simulink model "sampleModel1924_5_sub_sub"  (R2023a)
settings: Solver=VariableStepAuto  StartTime=0.0  StopTime=10.0  RelTol=1e-3
libraries: hdlsllib x5, simulink x2
settings Model: Creator=user1  LastModifiedBy=user1
settings OptimizationCC: BlockReduction=off  ConditionallyExecuteInputs=off

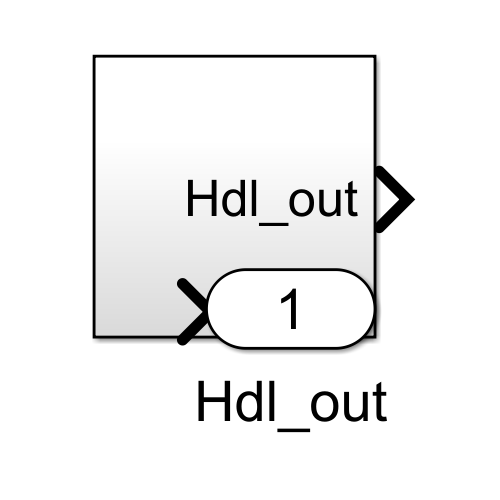
[thumbnail: Simulink's stored preview of the top-level diagram]
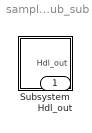
== system sampleModel1924_5_sub_sub ==
  Subsystem : Subsystem
  Hdl_out : Outport  OutDataTypeStr=uint8

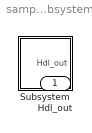
== system sampleModel1924_5_sub_sub/Subsystem ==
  Subsystem : Subsystem
  Hdl_out : Outport  OutDataTypeStr=uint8

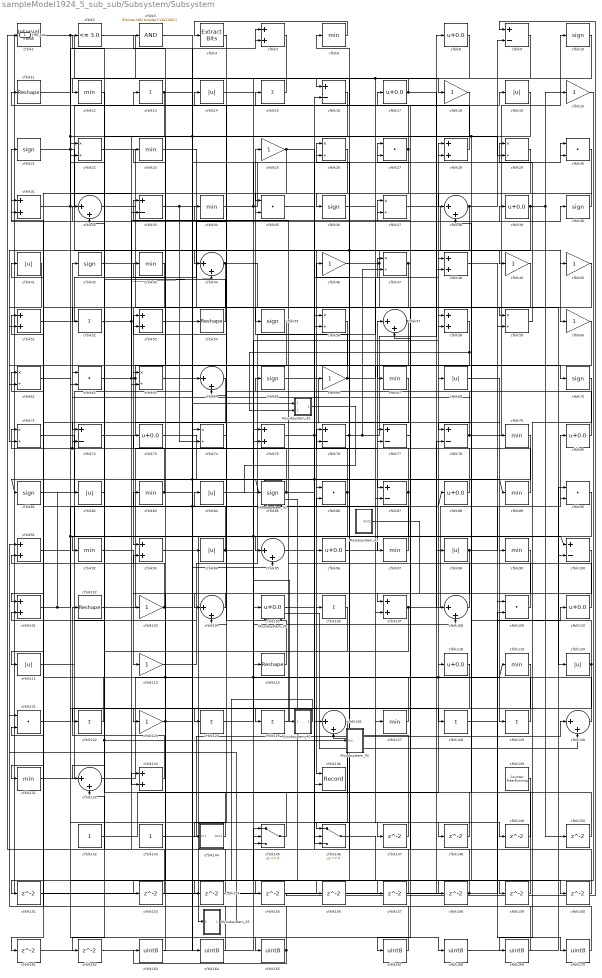
== system sampleModel1924_5_sub_sub/Subsystem/Subsystem ==
  Mysubsystem_25 : Subsystem  TreatAsAtomicUnit=on  RTWFcnName=Mysubsystem_25
      settings: RTWFcnNameOpts=User specified  RTWFileNameOpts=Use function name
  Mysubsystem_32 : Subsystem  TreatAsAtomicUnit=on  RTWFcnName=Mysubsystem_32
      settings: RTWFcnNameOpts=User specified  RTWFileNameOpts=Use function name
  Mysubsystem_39 : Subsystem  TreatAsAtomicUnit=on  RTWFcnName=Mysubsystem_39
      settings: RTWFcnNameOpts=User specified  RTWFileNameOpts=Use function name
  Mysubsystem_40 : Subsystem  TreatAsAtomicUnit=on  RTWFcnName=Mysubsystem_40
      settings: RTWFcnNameOpts=User specified  RTWFileNameOpts=Use function name
  Mysubsystem_41 : Subsystem  TreatAsAtomicUnit=on  RTWFcnName=Mysubsystem_41
      settings: RTWFcnNameOpts=User specified  RTWFileNameOpts=Use function name
  Mysubsystem_42 : Subsystem  TreatAsAtomicUnit=on  RTWFcnName=Mysubsystem_42
      settings: RTWFcnNameOpts=User specified  RTWFileNameOpts=Use function name
  Mysubsystem_43 : Subsystem  TreatAsAtomicUnit=on  RTWFcnName=Mysubsystem_43
      settings: RTWFcnNameOpts=User specified  RTWFileNameOpts=Use function name
  cfblk1 : hdlsllib/Logic and Bit Operations/Interval Test  IntervalClosedRight=on  uplimit=0.5  IntervalClosedLeft=on  lowlimit=-0.5  OutDataTypeStr=uint8
  cfblk{10,21,36,40,42,55,65,70,81,85} (10 alike) : Signum
  cfblk{9,16,33,72,76..78,87,100} (9 alike) : Sum  Inputs=+-  OutDataTypeStr=uint8
  cfblk{5,28,31,48,51,53,58,75,91,93,101,107,133} (13 alike) : Sum  OutDataTypeStr=uint8
  cfblk{11,54,102,115} (4 alike) : Reshape
  cfblk{18,20,25,46,49..50,60,66,103,113,123} (11 alike) : Gain  OutDataTypeStr=uint8
  cfblk{32,38,44,57,64,95,104,108,126,130,132} (11 alike) : Sum  Inputs=|++  OutDataTypeStr=uint8
  cfblk{8,17,39,73,80,88,96,105,110,118} (10 alike) : Bias  Bias=0.0  SaturateOnIntegerOverflow=off
  cfblk{13,15,52,106,122,124..125,128..129} (9 alike) : Sum  Inputs=+  OutDataTypeStr=uint8
  cfblk{27,30,35,62,86,90,109,121} (8 alike) : DotProduct  OutDataTypeStr=uint8
  cfblk{14,19,41,68,82,84,94,98,111,120} (10 alike) : Abs  OutDataTypeStr=uint8  SaturateOnIntegerOverflow=off
  cfblk{6,12,23,34,43,67,79,83,89,92,97,99,119,127,131} (15 alike) : MinMax  OutDataTypeStr=uint8
  cfblk136 : Record  FileSettingsInternal="{\"entries\":[{\"content\":{\"excelSettings\":{\"content\":{},\"type\":\"Streamout.ExcelSettings\"}},\"type\":\"Streamout.FileSettingStorage\",\"uuid\":\"\"}],\"packageUris\":[\"http:\\/\\/schema.mathworks.com\\/mf0\\/streamout_blocks\\/R2020a\"],\"version\":\"1.0\"}"  Layout=[1 1]  SignalsInternal="{\"entries\":[{\"content\":{\"signals\":[{\"content\":{\"blockPath\":[],\"dimensions\":[1],\"domain\":\"\",\"lineColor\":\"#a2142f\",\"plots\":[1],\"port\":1,\"signalID\":51994,\"signalName\":\"cfblk39\"},\"type\":\"RecordBlkView.Signal\",\"uuid\":\"\"},{\"content\":{\"blockPath\":[],\"dimensions\":[1],\"domain\":\"\",\"lineColor\":\"#139fff\",\"plots\":[1],\"port\":2,\"signalID\":51997,\"signalName\":\"cfblk44\"},\"type\":\"RecordBlkView.Signal\",\"uuid\":\"\"}]},\"type\":\"RecordBlkView.InputSignals\",\"uuid\":\"\"}],\"packageUris\":[\"http:\\/\\/schema.mathworks.com\\/mf0\\/streamout_blocks\\/R2020a\"],\"version\":\"1.0\"}"  VisualizationBindings="{\"xyplotplugin\":{\"info\":[{\"series\":[{\"bindingParametersList\":[{\"parameter\":\"X-Axis\",\"signalID\":51994,\"signalName\":\"cfblk39\"},{\"parameter\":\"Y-Axis\",\"signalID\":51997,\"signalName\":\"cfblk44\"}],\"seriesID\":57894}],\"subplotID\":1}]}}"  CompatibilityTag=XY  st=-1
  cfblk139 : hdlsllib/Sources/Counter Free-Running  NumBits=16  tsamp=-1
  cfblk142 : Constant  OutDataTypeStr=uint8  SampleTime=-1
  cfblk143 : Constant  OutDataTypeStr=uint8  SampleTime=-1
  cfblk144 : Subsystem
      settings: LibrarySourceBlock=|
      | hdlsllib/Ports &
      | Subsystems/Subsystem
  cfblk145 : Switch  OutDataTypeStr=uint8  SaturateOnIntegerOverflow=off  InputSameDT=off
  cfblk146 : Switch  OutDataTypeStr=uint8  SaturateOnIntegerOverflow=off  InputSameDT=off
  cfblk{147..151,153..162} (15 alike) : Delay  SampleTime=1
  cfblk{163..165,167..170} (7 alike) : DataTypeConversion  OutDataTypeStr=uint8  SaturateOnIntegerOverflow=off  RndMeth=Floor
  cfblk2 : hdlsllib/Logic and Bit Operations/Compare To Constant  relop=<=  const=3.0  OutDataTypeStr=uint8
  cfblk{22,26,29,37,47,56,59,61,63,71,74} (11 alike) : Product  Inputs=*/  OutDataTypeStr=uint8  RndMeth=Zero  SaturateOnIntegerOverflow=on
  cfblk3 : simulink/Logic and Bit Operations/Bitwise Operator  logicop=AND  UseBitMask=on  BitMask=bin2dec('11011001')  BitMaskRealWorld=Stored Integer
      settings: LibrarySourceBlock=|
      | hdlsllib/Logic and Bit
      | Operations/Bitwise
      | Operator
  cfblk4 : simulink/Logic and Bit Operations/Extract Bits  bitsToExtract=Upper half  numBits=8  bitIdxRange=[0 7]  outScalingMode=Preserve fixed-point scaling
      settings: LibrarySourceBlock=|
      | hdlsllib/Logic and Bit
      | Operations/Extract Bits
  Hdl_out : Outport  OutDataTypeStr=uint8
  wires:
  Mysubsystem_42/1(Out1) -> Mysubsystem_32/1(In1)
  Mysubsystem_41/1(Out1) -> cfblk104/1
  Mysubsystem_40/1(Out1) -> cfblk154/1
  Mysubsystem_39/1(Out1) -> cfblk130/2
  Mysubsystem_32/1(Out1) -> cfblk155/1
  Mysubsystem_25/1(Out1) -> cfblk121/1
  cfblk90/1 -> Mysubsystem_25/1(In1)
  cfblk170/1 -> cfblk91/2
  cfblk48/1 -> cfblk170/1
  cfblk169/1 -> cfblk91/1
  cfblk70/1 -> cfblk169/1
  cfblk168/1 -> cfblk90/1
  cfblk91/1 -> cfblk168/1
  cfblk167/1 -> cfblk121/2
  cfblk100/1 -> cfblk167/1
  cfblk165/1 -> cfblk163/1, cfblk43/1
  cfblk164/1 -> cfblk23/1
  cfblk3/1 -> cfblk164/1
  cfblk163/1 -> cfblk3/1
  cfblk162/1 -> cfblk64/1
  cfblk119/1 -> cfblk162/1
  cfblk161/1 -> cfblk145/1
  cfblk160/1 -> cfblk56/1
  cfblk146/1 -> cfblk160/1
  cfblk159/1 -> cfblk86/2
  cfblk158/1 -> cfblk57/2, Hdl_out/1
  cfblk157/1 -> cfblk76/2
  cfblk14/1 -> cfblk157/1
  cfblk156/1 -> cfblk78/2
  cfblk155/1 -> cfblk9/1
  cfblk154/1 -> cfblk133/1
  cfblk153/1 -> cfblk132/2
  cfblk151/1 -> cfblk109/2
  cfblk20/1 -> cfblk151/1
  cfblk150/1 -> cfblk38/2
  cfblk149/1 -> cfblk126/2
  cfblk95/1 -> cfblk149/1
  cfblk148/1 -> cfblk22/1
  cfblk36/1 -> cfblk148/1
  cfblk147/1 -> cfblk75/1
  cfblk8/1 -> cfblk22/2
  cfblk94/1 -> cfblk108/2, cfblk31/2
  cfblk12/1 -> cfblk72/1
  cfblk105/1 -> cfblk58/1
  cfblk71/1 -> cfblk108/1
  cfblk93/1 -> cfblk95/2
  cfblk125/1 -> cfblk65/1
  cfblk40/1 -> cfblk38/1
  cfblk98/1 -> cfblk90/2, cfblk153/1
  cfblk103/1 -> cfblk15/1, cfblk88/1, cfblk71/1
  cfblk88/1 -> cfblk26/1
  cfblk67/1 -> cfblk106/1
  cfblk56/1 -> cfblk75/2
  cfblk38/1 -> cfblk66/1, cfblk71/2, cfblk30/1
  cfblk57/1 -> cfblk97/1, cfblk27/1, cfblk61/2
  cfblk52/1 -> cfblk44/2, cfblk86/1
  cfblk5/1 -> cfblk44/1
  cfblk121/1 -> cfblk165/1
  cfblk82/1 -> cfblk2/1
  cfblk104/1 -> cfblk103/1
  cfblk85/1 -> cfblk73/1, cfblk47/1
  cfblk110/1 -> cfblk77/1
  cfblk60/1 -> cfblk78/1
  cfblk106/1 -> cfblk122/1
  cfblk79/1 -> cfblk81/1, cfblk146/2
  cfblk145/1 -> cfblk101/2
  cfblk30/1 -> cfblk35/1
  cfblk25/1 -> cfblk89/1, cfblk147/1, cfblk63/2
  cfblk64/1 -> cfblk111/1
  cfblk35/1 -> cfblk48/2
  cfblk2/1 -> cfblk115/1
  cfblk59/1 -> cfblk29/1
  cfblk61/1 -> cfblk99/1
  cfblk6/1 -> cfblk4/1
  cfblk81/1 -> cfblk37/2
  cfblk129/1 -> cfblk118/1
  cfblk84/1 -> Mysubsystem_40/1(In1), cfblk100/1
  cfblk101/1 -> cfblk83/1, cfblk82/1
  cfblk23/1 -> cfblk98/1
  cfblk19/1 -> cfblk63/1, cfblk158/1
  cfblk4/1 -> cfblk144/1(In1)
  cfblk33/1 -> cfblk120/1, cfblk74/2
  cfblk128/1 -> cfblk110/1
  cfblk99/1 -> cfblk123/1
  cfblk29/1 -> cfblk87/2
  cfblk11/1 -> cfblk33/2
  cfblk13/1 -> cfblk95/1, cfblk52/1
  cfblk9/1 -> cfblk107/2, cfblk146/1
  cfblk15/1 -> cfblk12/1
  cfblk10/1 -> cfblk36/1
  cfblk83/1 -> cfblk85/1, cfblk27/2, cfblk41/1, cfblk72/2
  cfblk18/1 -> cfblk133/2
  cfblk1/1 -> Mysubsystem_42/1(In1), cfblk29/2, cfblk145/3, cfblk18/1
  cfblk115/1 -> cfblk53/2
  cfblk75/1 -> cfblk40/1, cfblk77/2
  cfblk65/1 -> cfblk127/1
  cfblk41/1 -> cfblk51/2
  cfblk113/1 -> cfblk48/1
  cfblk26/1 -> cfblk62/2
  cfblk130/1 -> cfblk68/1, cfblk46/1
  cfblk62/1 -> cfblk67/1, cfblk105/1, cfblk35/2
  cfblk109/1 -> cfblk33/1
  cfblk76/1 -> cfblk8/1, cfblk47/2, cfblk26/2
  cfblk16/1 -> cfblk124/1
  cfblk42/1 -> cfblk126/1
  cfblk126/1 -> cfblk145/2
  cfblk124/1 -> cfblk119/1, cfblk58/2
  cfblk46/1 -> cfblk50/1, cfblk59/1
  cfblk87/1 -> cfblk92/1, cfblk31/1
  cfblk77/1 -> cfblk107/1
  cfblk111/1 -> cfblk16/2
  cfblk32/1 -> cfblk109/1
  cfblk22/1 -> cfblk56/2
  cfblk27/1 -> cfblk11/1, cfblk161/1
  cfblk122/1 -> cfblk51/1
  cfblk49/1 -> cfblk87/1
  cfblk143/1 -> cfblk130/1
  cfblk51/1 -> cfblk39/1
  cfblk108/1 -> cfblk37/1
  cfblk127/1 -> cfblk53/1, cfblk61/1
  cfblk54/1 -> cfblk32/2
  cfblk73/1 -> cfblk96/1
  cfblk43/1 -> cfblk93/1
  cfblk74/1 -> cfblk14/1
  cfblk120/1 -> cfblk62/1, cfblk156/1
  cfblk139/1 -> cfblk1/1
  cfblk37/1 -> cfblk49/1
  cfblk53/1 -> cfblk94/1
  cfblk50/1 -> cfblk101/1
  cfblk118/1 -> cfblk125/1
  cfblk96/1 -> cfblk57/1
  cfblk102/1 -> cfblk76/1
  cfblk72/1 -> cfblk79/1
  cfblk144/1(Out1) -> cfblk13/1
  cfblk44/1 -> Mysubsystem_43/1(In1), cfblk132/1, cfblk136/2
  cfblk34/1 -> cfblk9/2, cfblk30/2
  cfblk28/1 -> cfblk6/1
  cfblk80/1 -> cfblk28/2
  cfblk39/1 -> cfblk20/1, cfblk150/1, cfblk136/1
  cfblk58/1 -> Mysubsystem_42/2(In2), cfblk131/1
  cfblk123/1 -> cfblk74/1, cfblk93/2
  cfblk47/1 -> cfblk55/1, cfblk17/1
  cfblk68/1 -> cfblk129/1
  cfblk86/1 -> cfblk32/1, cfblk104/2
  cfblk142/1 -> cfblk28/1
  cfblk55/1 -> cfblk64/2
  cfblk21/1 -> cfblk100/2, cfblk128/1, cfblk60/1
  cfblk133/1 -> cfblk102/1
  cfblk78/1 -> cfblk10/1, cfblk34/1
  cfblk63/1 -> cfblk5/1
  cfblk107/1 -> cfblk80/1, cfblk146/3
  cfblk66/1 -> cfblk25/1, cfblk70/1
  cfblk89/1 -> cfblk42/1
  cfblk97/1 -> cfblk21/1
  cfblk132/1 -> cfblk54/1
  cfblk92/1 -> cfblk113/1
  cfblk131/1 -> cfblk84/1
  cfblk17/1 -> cfblk16/1, cfblk59/2
  cfblk31/1 -> cfblk19/1, cfblk5/2, cfblk159/1

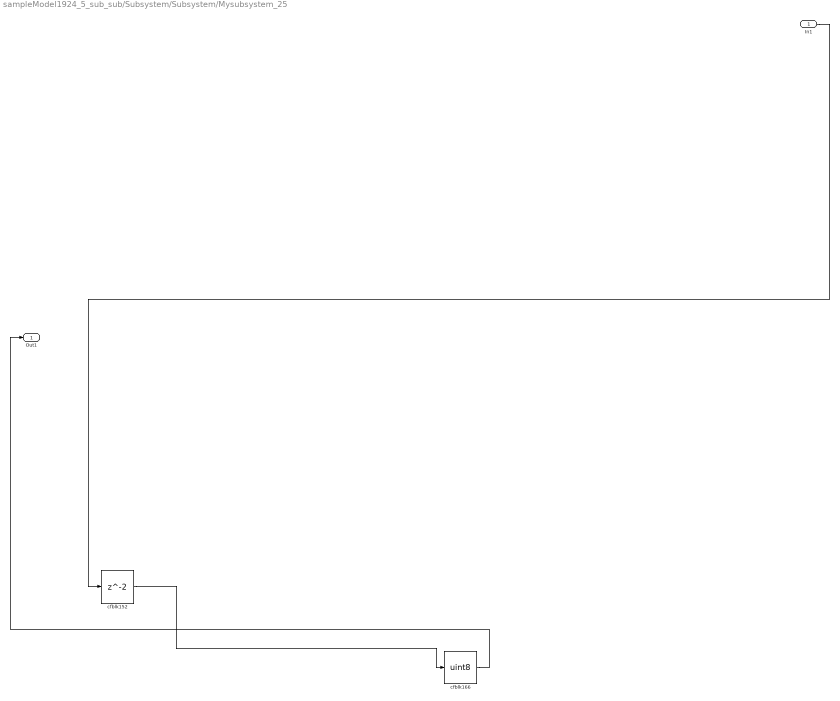
== system sampleModel1924_5_sub_sub/Subsystem/Subsystem/Mysubsystem_25 ==
  In1 : Inport
  cfblk152 : Delay  SampleTime=1
  cfblk166 : DataTypeConversion  OutDataTypeStr=uint8  SaturateOnIntegerOverflow=off  RndMeth=Floor
  Out1 : Outport
  wires:
  cfblk152/1 -> cfblk166/1
  In1/1 -> cfblk152/1
  cfblk166/1 -> Out1/1

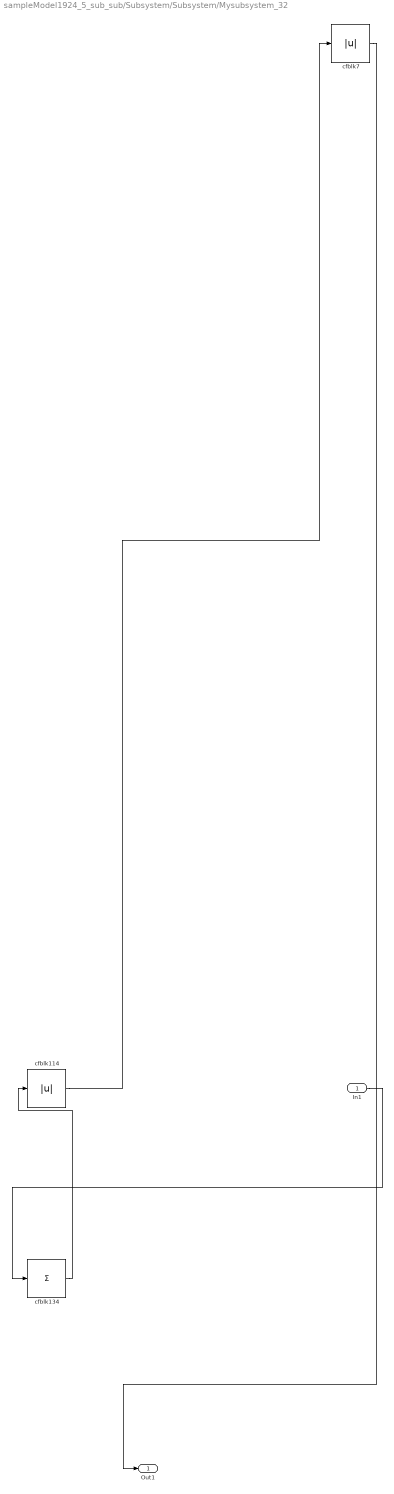
== system sampleModel1924_5_sub_sub/Subsystem/Subsystem/Mysubsystem_32 ==
  In1 : Inport
  cfblk114 : Abs  SaturateOnIntegerOverflow=off
  cfblk134 : Sum  Inputs=+
  cfblk7 : Abs  SaturateOnIntegerOverflow=off
  Out1 : Outport
  wires:
  cfblk7/1 -> Out1/1
  cfblk114/1 -> cfblk7/1
  cfblk134/1 -> cfblk114/1
  In1/1 -> cfblk134/1

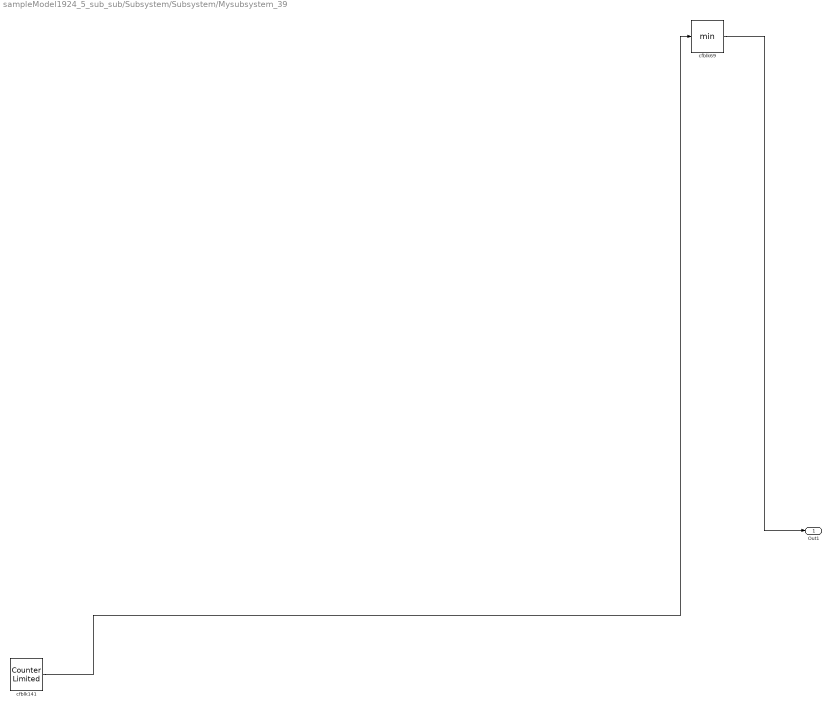
== system sampleModel1924_5_sub_sub/Subsystem/Subsystem/Mysubsystem_39 ==
  cfblk141 : hdlsllib/Sources/Counter Limited  uplimit=7  tsamp=-1
  cfblk69 : MinMax
  Out1 : Outport
  wires:
  cfblk69/1 -> Out1/1
  cfblk141/1 -> cfblk69/1

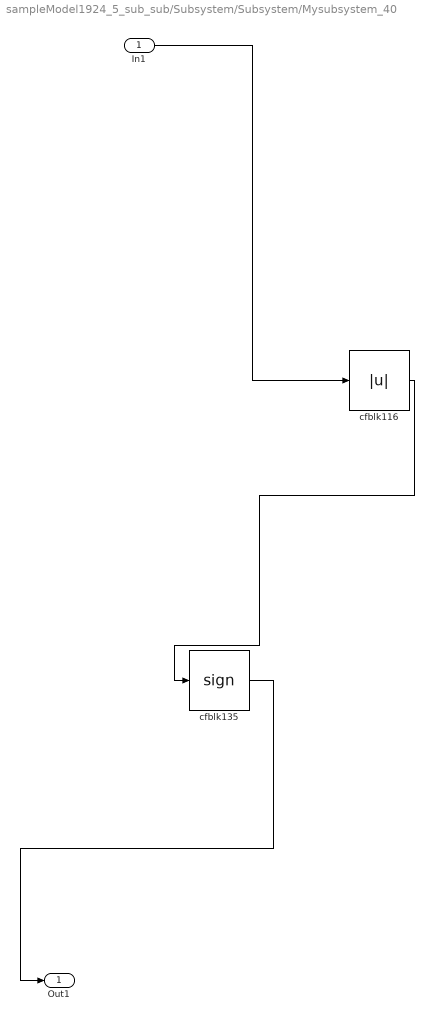
== system sampleModel1924_5_sub_sub/Subsystem/Subsystem/Mysubsystem_40 ==
  In1 : Inport
  cfblk116 : Abs  SaturateOnIntegerOverflow=off
  cfblk135 : Signum
  Out1 : Outport
  wires:
  cfblk116/1 -> cfblk135/1
  cfblk135/1 -> Out1/1
  In1/1 -> cfblk116/1

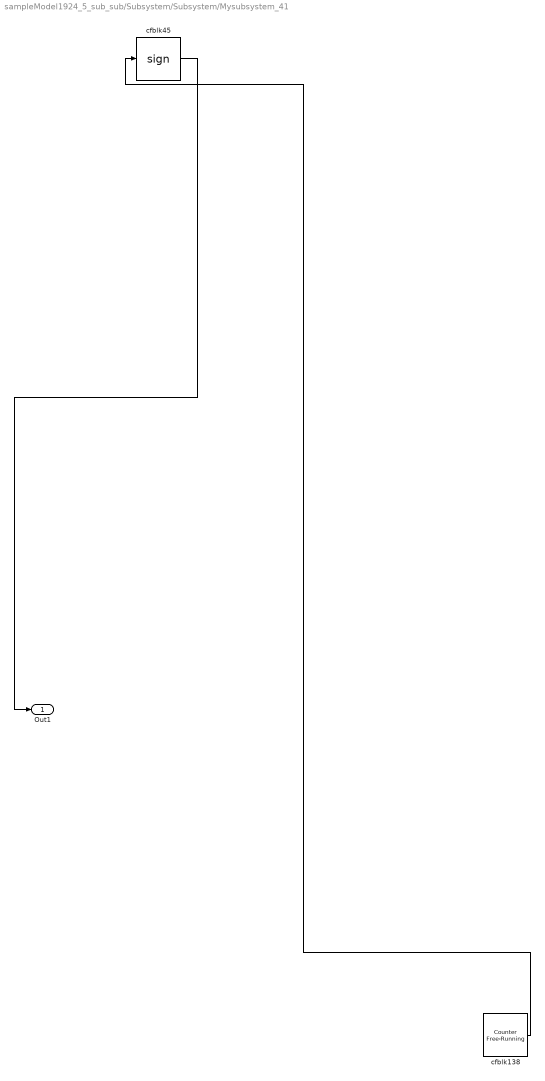
== system sampleModel1924_5_sub_sub/Subsystem/Subsystem/Mysubsystem_41 ==
  cfblk138 : hdlsllib/Sources/Counter Free-Running  NumBits=16  tsamp=-1
  cfblk45 : Signum
  Out1 : Outport
  wires:
  cfblk138/1 -> cfblk45/1
  cfblk45/1 -> Out1/1

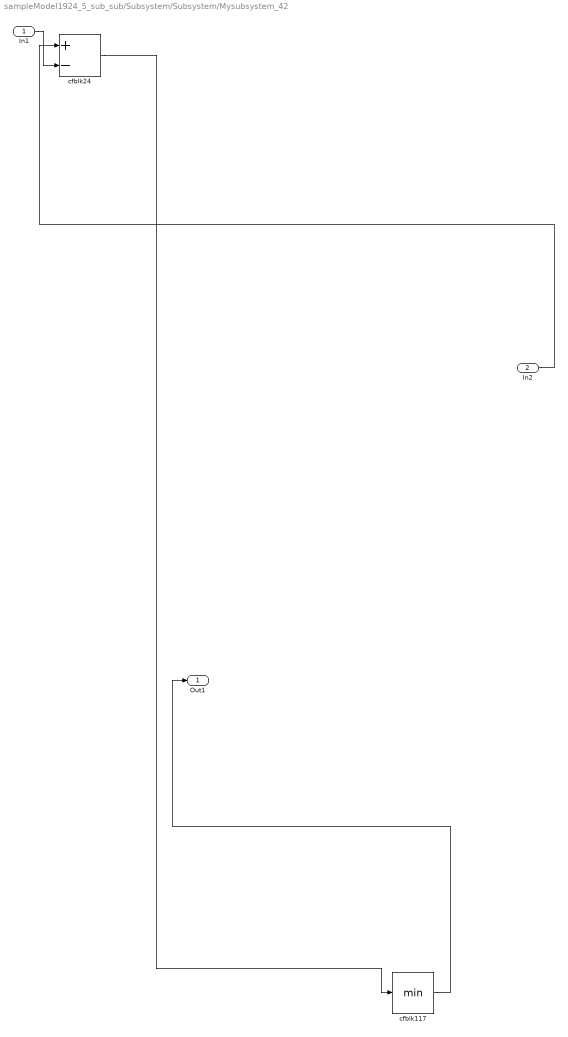
== system sampleModel1924_5_sub_sub/Subsystem/Subsystem/Mysubsystem_42 ==
  In1 : Inport
  In2 : Inport  Port=2
  cfblk117 : MinMax
  cfblk24 : Sum  Inputs=+-
  Out1 : Outport
  wires:
  In2/1 -> cfblk24/1
  cfblk24/1 -> cfblk117/1
  cfblk117/1 -> Out1/1
  In1/1 -> cfblk24/2

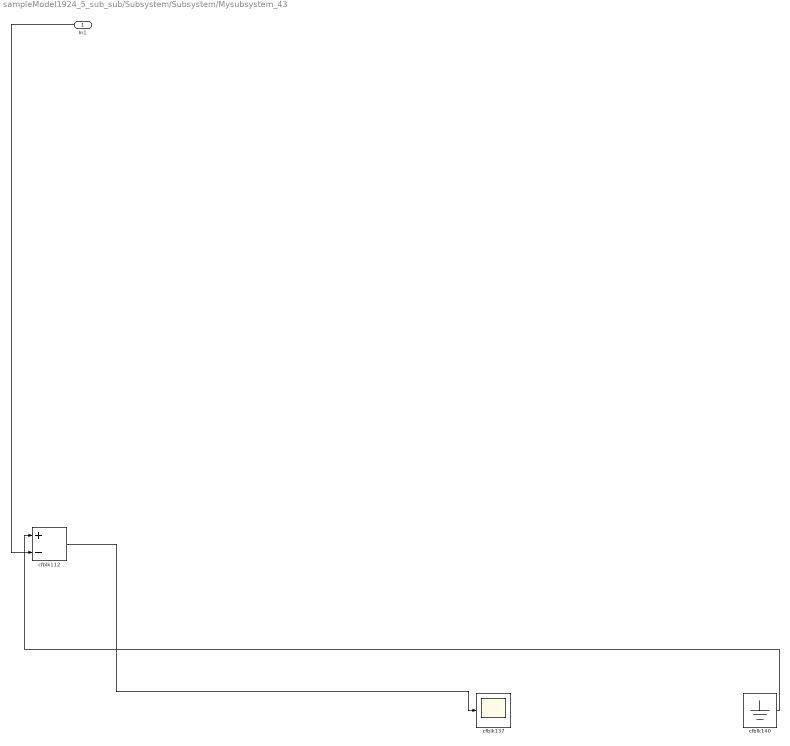
== system sampleModel1924_5_sub_sub/Subsystem/Subsystem/Mysubsystem_43 ==
  In1 : Inport
  cfblk112 : Sum  Inputs=+-
  cfblk137 : Scope
  cfblk140 : Ground
  wires:
  cfblk140/1 -> cfblk112/1
  cfblk112/1 -> cfblk137/1
  In1/1 -> cfblk112/2

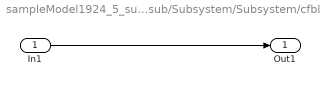
== system sampleModel1924_5_sub_sub/Subsystem/Subsystem/cfblk144 ==
  In1 : Inport
  Out1 : Outport
  wires:
  In1/1 -> Out1/1
